simulink model "automata_learning"  (R2022a)
(part 6 of 10)

0.1781599223613739 * x2 - 0.022882848978042603) - 1.0) / (exp(0.6783225536346436 * x1 + 0.1781599223613739 * x2 - 0.022882848978042603) + 1.0) + 0.600735068321228 * (exp(0.485967755317688 * x2 - 1.1853820085525513 * x1 + 0.018565522506833076) - 1.0) / (exp(0.485967755317688 * x2 - 1.1853820085525513 * x1 + 0.018565522506833076) + 1.0) + 0.07953598350286484 * (exp(1.4361170530319214 * x1 - 0.5143741369247437 * x2 + 0.003782355459406972) - 1.0) / (exp(1.4361170530319214 * x1 - 0.5143741369247437 * x2 + 0.003782355459406972) + 1.0) - 0.3439609110355377 * (exp(1.0996636152267456 * x1 - 0.4135805368423462 * x2 + 0.20608894526958466) - 1.0) / (exp(1.0996636152267456 * x1 - 0.4135805368423462 * x2 + 0.20608894526958466) + 1.0) - 0.26753464341163635 * (exp(1.101186752319336 * x1 + 0.23448167741298676 * x2 - 0.7151159048080444) - 1.0) / (exp(1.101186752319336 * x1 + 0.23448167741298676 * x2 - 0.7151159048080444) + 1.0) - 0.33746933937072754 * (exp(0.2064213752746582 * x1 + 0.17808765172958374 * x2 - 0.17820464074611664) - 1.0) / (exp(0.2064213752746582 * x1 + 0.17808765172958374 * x2 - 0.17820464074611664) + 1.0) + 0.7188074588775635 * (exp(0.8331294059753418 * x1 + 0.364244282245636 * x2 - 0.19144871830940247) - 1.0) / (exp(0.8331294059753418 * x1 + 0.364244282245636 * x2 - 0.19144871830940247) + 1.0) + 0.48850470781326294 * (exp(0.4359053075313568 * x1 + 0.912689745426178 * x2 + 0.2776009142398834) - 1.0) / (exp(0.4359053075313568 * x1 + 0.912689745426178 * x2 + 0.2776009142398834) + 1.0) - 0.3132037818431854 * (exp(0.4313433766365051 * x1 + 0.24489279091358185 * x2 - 0.033217817544937134) - 1.0) / (exp(0.4313433766365051 * x1 + 0.24489279091358185 * x2 - 0.033217817544937134) + 1.0) + 0.5981374979019165 * (exp(0.3509118854999542 * x1 - 0.9669473171234131 * x2 + 0.38815683126449585) - 1.0) / (exp(0.3509118854999542 * x1 - 0.9669473171234131 * x2 + 0.38815683126449585) + 1.0) + 0.47281572222709656 * (exp(0.8456477522850037 * x1 - 0.048582736402750015 * x2 + 0.05466446280479431) - 1.0) / (exp(0.8456477522850037 * x1 - 0.048582736402750015 * x2 + 0.05466446280479431) + 1.0) - 0.7066691517829895 * (exp(0.37150701880455017 * x1 - 0.23563559353351593 * x2 + 0.41328972578048706) - 1.0) / (exp(0.37150701880455017 * x1 - 0.23563559353351593 * x2 + 0.41328972578048706) + 1.0) - 0.5022667050361633 * (exp(1.5675164461135864 * x1 + 0.05015593022108078 * x2 + 0.23397907614707947) - 1.0) / (exp(1.5675164461135864 * x1 + 0.05015593022108078 * x2 + 0.23397907614707947) + 1.0) + 0.6585901379585266 * (exp(0.66331547498703 * x1 + 0.4469437301158905 * x2 + 0.06243124231696129) - 1.0) / (exp(0.66331547498703 * x1 + 0.4469437301158905 * x2 + 0.06243124231696129) + 1.0) + 0.12011811137199402) + 1.0) - 0.2208395153284073 * (exp(0.36608901619911194 * (exp(0.8134481906890869 * x1 + 0.9884344339370728 * x2 - 0.4219200313091278) - 1.0) / (exp(0.8134481906890869 * x1 + 0.9884344339370728 * x2 - 0.4219200313091278) + 1.0) - 0.7763866186141968 * (exp(0.4392474293708801 * x1 - 0.48300591111183167 * x2 + 0.1989256739616394) - 1.0) / (exp(0.4392474293708801 * x1 - 0.48300591111183167 * x2 + 0.1989256739616394) + 1.0) + 0.3814668357372284 * (exp(0.047009728848934174 * x2 - 1.010794997215271 * x1 + 0.010623830370604992) - 1.0) / (exp(0.047009728848934174 * x2 - 1.010794997215271 * x1 + 0.010623830370604992) + 1.0) + 0.550957977771759 * (exp(0.8894705772399902 * x1 - 1.0577815771102905 * x2 + 0.6941524744033813) - 1.0) / (exp(0.8894705772399902 * x1 - 1.0577815771102905 * x2 + 0.6941524744033813) + 1.0) - 0.42258381843566895 * (exp(0.8751505613327026 * x1 + 0.041782353073358536 * x2 + 0.14423272013664246) - 1.0) / (exp(0.8751505613327026 * x1 + 0.041782353073358536 * x2 + 0.14423272013664246) + 1.0) - 0.33416351675987244 * (exp(0.1809358298778534 * x2 - 1.0878992080688477 * x1 + 0.21376754343509674) - 1.0) / (exp(0.1809358298778534 * x2 - 1.0878992080688477 * x1 + 0.21376754343509674) + 1.0) - 0.5293717384338379 * (exp(0.6783225536346436 * x1 + 0.1781599223613739 * x2 - 0.022882848978042603) - 1.0) / (exp(0.6783225536346436 * x1 + 0.1781599223613739 * x2 - 0.022882848978042603) + 1.0) + 0.16978411376476288 * (exp(0.485967755317688 * x2 - 1.1853820085525513 * x1 + 0.018565522506833076) - 1.0) / (exp(0.485967755317688 * x2 - 1.1853820085525513 * x1 + 0.018565522506833076) + 1.0) - 0.07960239797830582 * (exp(1.4361170530319214 * x1 - 0.5143741369247437 * x2 + 0.003782355459406972) - 1.0) / (exp(1.4361170530319214 * x1 - 0.5143741369247437 * x2 + 0.003782355459406972) + 1.0) + 0.3012309670448303 * (exp(1.0996636152267456 * x1 - 0.4135805368423462 * x2 + 0.20608894526958466) - 1.0) / (exp(1.0996636152267456 * x1 - 0.4135805368423462 * x2 + 0.20608894526958466) + 1.0) + 0.001827016705647111 * (exp(1.101186752319336 * x1 + 0.23448167741298676 * x2 - 0.7151159048080444) - 1.0) / (exp(1.101186752319336 * x1 + 0.23448167741298676 * x2 - 0.7151159048080444) + 1.0) + 0.6800966262817383 * (exp(0.2064213752746582 * x1 + 0.17808765172958374 * x2 - 0.17820464074611664) - 1.0) / (exp(0.2064213752746582 * x1 + 0.17808765172958374 * x2 - 0.17820464074611664) + 1.0) + 0.3445820212364197 * (exp(0.8331294059753418 * x1 + 0.364244282245636 * x2 - 0.19144871830940247) - 1.0) / (exp(0.8331294059753418 * x1 + 0.364244282245636 * x2 - 0.19144871830940247) + 1.0) + 0.33697742223739624 * (exp(0.4359053075313568 * x1 + 0.912689745426178 * x2 + 0.2776009142398834) - 1.0) / (exp(0.4359053075313568 * x1 + 0.912689745426178 * x2 + 0.2776009142398834) + 1.0) + 0.6987252831459045 * (exp(0.4313433766365051 * x1 + 0.24489279091358185 * x2 - 0.033217817544937134) - 1.0) / (exp(0.4313433766365051 * x1 + 0.24489279091358185 * x2 - 0.033217817544937134) + 1.0) - 0.700903058052063 * (exp(0.3509118854999542 * x1 - 0.9669473171234131 * x2 + 0.38815683126449585) - 1.0) / (exp(0.3509118854999542 * x1 - 0.9669473171234131 * x2 + 0.38815683126449585) + 1.0) - 0.48154786229133606 * (exp(0.8456477522850037 * x1 - 0.048582736402750015 * x2 + 0.05466446280479431) - 1.0) / (exp(0.8456477522850037 * x1 - 0.048582736402750015 * x2 + 0.05466446280479431) + 1.0) - 0.6501414775848389 * (exp(0.37150701880455017 * x1 - 0.23563559353351593 * x2 + 0.41328972578048706) - 1.0) / (exp(0.37150701880455017 * x1 - 0.23563559353351593 * x2 + 0.41328972578048706) + 1.0) - 0.5015138387680054 * (exp(1.5675164461135864 * x1 + 0.05015593022108078 * x2 + 0.23397907614707947) - 1.0) / (exp(1.5675164461135864 * x1 + 0.05015593022108078 * x2 + 0.23397907614707947) + 1.0) - 0.13284653425216675 * (exp(0.66331547498703 * x1 + 0.4469437301158905 * x2 + 0.06243124231696129) - 1.0) / (exp(0.66331547498703 * x1 + 0.4469437301158905 * x2 + 0.06243124231696129) + 1.0) + 0.036147914826869965) - 1.0) / (exp(0.36608901619911194 * (exp(0.8134481906890869 * x1 + 0.9884344339370728 * x2 - 0.4219200313091278) - 1.0) / (exp(0.8134481906890869 * x1 + 0.9884344339370728 * x2 - 0.4219200313091278) + 1.0) - 0.7763866186141968 * (exp(0.4392474293708801 * x1 - 0.48300591111183167 * x2 + 0.1989256739616394) - 1.0) / (exp(0.4392474293708801 * x1 - 0.48300591111183167 * x2 + 0.1989256739616394) + 1.0) + 0.3814668357372284 * (exp(0.047009728848934174 * x2 - 1.010794997215271 * x1 + 0.010623830370604992) - 1.0) / (exp(0.047009728848934174 * x2 - 1.010794997215271 * x1 + 0.010623830370604992) + 1.0) + 0.550957977771759 * (exp(0.8894705772399902 * x1 - 1.0577815771102905 * x2 + 0.6941524744033813) - 1.0) / (exp(0.8894705772399902 * x1 - 1.0577815771102905 * x2 + 0.6941524744033813) + 1.0) - 0.42258381843566895 * (exp(0.8751505613327026 * x1 + 0.041782353073358536 * x2 + 0.14423272013664246) - 1.0) / (exp(0.8751505613327026 * x1 + 0.041782353073358536 * x2 + 0.14423272013664246) + 1.0) - 0.33416351675987244 * (exp(0.1809358298778534 * x2 - 1.0878992080688477 * x1 + 0.21376754343509674) - 1.0) / (exp(0.1809358298778534 * x2 - 1.0878992080688477 * x1 + 0.21376754343509674) + 1.0) - 0.5293717384338379 * (exp(0.6783225536346436 * x1 + 0.1781599223613739 * x2 - 0.022882848978042603) - 1.0) / (exp(0.6783225536346436 * x1 + 0.1781599223613739 * x2 - 0.022882848978042603) + 1.0) + 0.16978411376476288 * (exp(0.485967755317688 * x2 - 1.1853820085525513 * x1 + 0.018565522506833076) - 1.0) / (exp(0.485967755317688 * x2 - 1.1853820085525513 * x1 + 0.018565522506833076) + 1.0) - 0.07960239797830582 * (exp(1.4361170530319214 * x1 - 0.5143741369247437 * x2 + 0.003782355459406972) - 1.0) / (exp(1.4361170530319214 * x1 - 0.5143741369247437 * x2 + 0.003782355459406972) + 1.0) + 0.3012309670448303 * (exp(1.0996636152267456 * x1 - 0.4135805368423462 * x2 + 0.20608894526958466) - 1.0) / (exp(1.0996636152267456 * x1 - 0.4135805368423462 * x2 + 0.20608894526958466) + 1.0) + 0.001827016705647111 * (exp(1.101186752319336 * x1 + 0.23448167741298676 * x2 - 0.7151159048080444) - 1.0) / (exp(1.101186752319336 * x1 + 0.23448167741298676 * x2 - 0.7151159048080444) + 1.0) + 0.6800966262817383 * (exp(0.2064213752746582 * x1 + 0.17808765172958374 * x2 - 0.17820464074611664) - 1.0) / (exp(0.2064213752746582 * x1 + 0.17808765172958374 * x2 - 0.17820464074611664) + 1.0) + 0.3445820212364197 * (exp(0.8331294059753418 * x1 + 0.364244282245636 * x2 - 0.19144871830940247) - 1.0) / (exp(0.8331294059753418 * x1 + 0.364244282245636 * x2 - 0.19144871830940247) + 1.0) + 0.33697742223739624 * (exp(0.4359053075313568 * x1 + 0.912689745426178 * x2 + 0.2776009142398834) - 1.0) / (exp(0.4359053075313568 * x1 + 0.912689745426178 * x2 + 0.2776009142398834) + 1.0) + 0.6987252831459045 * (exp(0.4313433766365051 * x1 + 0.24489279091358185 * x2 - 0.033217817544937134) - 1.0) / (exp(0.4313433766365051 * x1 + 0.24489279091358185 * x2 - 0.033217817544937134) + 1.0) - 0.700903058052063 * (exp(0.3509118854999542 * x1 - 0.9669473171234131 * x2 + 0.38815683126449585) - 1.0) / (exp(0.3509118854999542 * x1 - 0.9669473171234131 * x2 + 0.38815683126449585) + 1.0) - 0.48154786229133606 * (exp(0.8456477522850037 * x1 - 0.048582736402750015 * x2 + 0.05466446280479431) - 1.0) / (exp(0.8456477522850037 * x1 - 0.048582736402750015 * x2 + 0.05466446280479431) + 1.0) - 0.6501414775848389 * (exp(0.37150701880455017 * x1 - 0.23563559353351593 * x2 + 0.41328972578048706) - 1.0) / (exp(0.37150701880455017 * x1 - 0.23563559353351593 * x2 + 0.41328972578048706) + 1.0) - 0.5015138387680054 * (exp(1.5675164461135864 * x1 + 0.05015593022108078 * x2 + 0.23397907614707947) - 1.0) / (exp(1.5675164461135864 * x1 + 0.05015593022108078 * x2 + 0.23397907614707947) + 1.0) - 0.13284653425216675 * (exp(0.66331547498703 * x1 + 0.4469437301158905 * x2 + 0.06243124231696129) - 1.0) / (exp(0.66331547498703 * x1 + 0.4469437301158905 * x2 + 0.06243124231696129) + 1.0) + 0.036147914826869965) + 1.0) + 0.5369366407394409 * (exp(0.41898313164711 * (exp(0.4392474293708801 * x1 - 0.48300591111183167 * x2 + 0.1989256739616394) - 1.0) / (exp(0.4392474293708801 * x1 - 0.48300591111183167 * x2 + 0.1989256739616394) + 1.0) + 0.5099337100982666 * (exp(0.8134481906890869 * x1 + 0.9884344339370728 * x2 - 0.4219200313091278) - 1.0) / (exp(0.8134481906890869 * x1 + 0.9884344339370728 * x2 - 0.4219200313091278) + 1.0) - 0.1566210687160492 * (exp(0.047009728848934174 * x2 - 1.010794997215271 * x1 + 0.010623830370604992) - 1.0) / (exp(0.047009728848934174 * x2 - 1.010794997215271 * x1 + 0.010623830370604992) + 1.0) + 0.6093736886978149 * (exp(0.8894705772399902 * x1 - 1.0577815771102905 * x2 + 0.6941524744033813) - 1.0) / (exp(0.8894705772399902 * x1 - 1.0577815771102905 * x2 + 0.6941524744033813) + 1.0) - 0.6370351910591125 * (exp(0.8751505613327026 * x1 + 0.041782353073358536 * x2 + 0.14423272013664246) - 1.0) / (exp(0.8751505613327026 * x1 + 0.041782353073358536 * x2 + 0.14423272013664246) + 1.0) + 0.0998457819223404 * (exp(0.1809358298778534 * x2 - 1.0878992080688477 * x1 + 0.21376754343509674) - 1.0) / (exp(0.1809358298778534 * x2 - 1.0878992080688477 * x1 + 0.21376754343509674) + 1.0) + 0.7771844863891602 * (exp(0.6783225536346436 * x1 + 0.1781599223613739 * x2 - 0.022882848978042603) - 1.0) / (exp(0.6783225536346436 * x1 + 0.1781599223613739 * x2 - 0.022882848978042603) + 1.0) + 0.7646798491477966 * (exp(0.485967755317688 * x2 - 1.1853820085525513 * x1 + 0.018565522506833076) - 1.0) / (exp(0.485967755317688 * x2 - 1.1853820085525513 * x1 + 0.018565522506833076) + 1.0) - 0.14706474542617798 * (exp(1.4361170530319214 * x1 - 0.5143741369247437 * x2 + 0.003782355459406972) - 1.0) / (exp(1.4361170530319214 * x1 - 0.5143741369247437 * x2 + 0.003782355459406972) + 1.0) + 0.44270166754722595 * (exp(1.0996636152267456 * x1 - 0.4135805368423462 * x2 + 0.20608894526958466) - 1.0) / (exp(1.0996636152267456 * x1 - 0.4135805368423462 * x2 + 0.20608894526958466) + 1.0) + 0.05599430948495865 * (exp(1.101186752319336 * x1 + 0.23448167741298676 * x2 - 0.7151159048080444) - 1.0) / (exp(1.101186752319336 * x1 + 0.23448167741298676 * x2 - 0.7151159048080444) + 1.0) - 0.4630465507507324 * (exp(0.2064213752746582 * x1 + 0.17808765172958374 * x2 - 0.17820464074611664) - 1.0) / (exp(0.2064213752746582 * x1 + 0.17808765172958374 * x2 - 0.17820464074611664) + 1.0) + 0.8380157351493835 * (exp(0.8331294059753418 * x1 + 0.364244282245636 * x2 - 0.19144871830940247) - 1.0) / (exp(0.8331294059753418 * x1 + 0.364244282245636 * x2 - 0.19144871830940247) + 1.0) + 0.12685304880142212 * (exp(0.4359053075313568 * x1 + 0.912689745426178 * x2 + 0.2776009142398834) - 1.0) / (exp(0.4359053075313568 * x1 + 0.912689745426178 * x2 + 0.2776009142398834) + 1.0) - 0.704443097114563 * (exp(0.4313433766365051 * x1 + 0.24489279091358185 * x2 - 0.033217817544937134) - 1.0) / (exp(0.4313433766365051 * x1 + 0.24489279091358185 * x2 - 0.033217817544937134) + 1.0) + 0.23543411493301392 * (exp(0.3509118854999542 * x1 - 0.9669473171234131 * x2 + 0.38815683126449585) - 1.0) / (exp(0.3509118854999542 * x1 - 0.9669473171234131 * x2 + 0.38815683126449585) + 1.0) - 0.16425514221191406 * (exp(0.8456477522850037 * x1 - 0.048582736402750015 * x2 + 0.05466446280479431) - 1.0) / (exp(0.8456477522850037 * x1 - 0.048582736402750015 * x2 + 0.05466446280479431) + 1.0) + 0.33761852979660034 * (exp(0.37150701880455017 * x1 - 0.23563559353351593 * x2 + 0.41328972578048706) - 1.0) / (exp(0.37150701880455017 * x1 - 0.23563559353351593 * x2 + 0.41328972578048706) + 1.0) - 0.23770417273044586 * (exp(1.5675164461135864 * x1 + 0.05015593022108078 * x2 + 0.23397907614707947) - 1.0) / (exp(1.5675164461135864 * x1 + 0.05015593022108078 * x2 + 0.23397907614707947) + 1.0) + 0.6810302138328552 * (exp(0.66331547498703 * x1 + 0.4469437301158905 * x2 + 0.06243124231696129) - 1.0) / (exp(0.66331547498703 * x1 + 0.4469437301158905 * x2 + 0.06243124231696129) + 1.0) + 0.16052111983299255) - 1.0) / (exp(0.41898313164711 * (exp(0.4392474293708801 * x1 - 0.48300591111183167 * x2 + 0.1989256739616394) - 1.0) / (exp(0.4392474293708801 * x1 - 0.48300591111183167 * x2 + 0.1989256739616394) + 1.0) + 0.5099337100982666 * (exp(0.8134481906890869 * x1 + 0.9884344339370728 * x2 - 0.4219200313091278) - 1.0) / (exp(0.8134481906890869 * x1 + 0.9884344339370728 * x2 - 0.4219200313091278) + 1.0) - 0.1566210687160492 * (exp(0.047009728848934174 * x2 - 1.010794997215271 * x1 + 0.010623830370604992) - 1.0) / (exp(0.047009728848934174 * x2 - 1.010794997215271 * x1 + 0.010623830370604992) + 1.0) + 0.6093736886978149 * (exp(0.8894705772399902 * x1 - 1.0577815771102905 * x2 + 0.6941524744033813) - 1.0) / (exp(0.8894705772399902 * x1 - 1.0577815771102905 * x2 + 0.6941524744033813) + 1.0) - 0.6370351910591125 * (exp(0.8751505613327026 * x1 + 0.041782353073358536 * x2 + 0.14423272013664246) - 1.0) / (exp(0.8751505613327026 * x1 + 0.041782353073358536 * x2 + 0.14423272013664246) + 1.0) + 0.0998457819223404 * (exp(0.1809358298778534 * x2 - 1.0878992080688477 * x1 + 0.21376754343509674) - 1.0) / (exp(0.1809358298778534 * x2 - 1.0878992080688477 * x1 + 0.21376754343509674) + 1.0) + 0.7771844863891602 * (exp(0.6783225536346436 * x1 + 0.1781599223613739 * x2 - 0.022882848978042603) - 1.0) / (exp(0.6783225536346436 * x1 + 0.1781599223613739 * x2 - 0.022882848978042603) + 1.0) + 0.7646798491477966 * (exp(0.485967755317688 * x2 - 1.1853820085525513 * x1 + 0.018565522506833076) - 1.0) / (exp(0.485967755317688 * x2 - 1.1853820085525513 * x1 + 0.018565522506833076) + 1.0) - 0.14706474542617798 * (exp(1.4361170530319214 * x1 - 0.5143741369247437 * x2 + 0.003782355459406972) - 1.0) / (exp(1.4361170530319214 * x1 - 0.5143741369247437 * x2 + 0.003782355459406972) + 1.0) + 0.44270166754722595 * (exp(1.0996636152267456 * x1 - 0.4135805368423462 * x2 + 0.20608894526958466) - 1.0) / (exp(1.0996636152267456 * x1 - 0.4135805368423462 * x2 + 0.20608894526958466) + 1.0) + 0.05599430948495865 * (exp(1.101186752319336 * x1 + 0.23448167741298676 * x2 - 0.7151159048080444) - 1.0) / (exp(1.101186752319336 * x1 + 0.23448167741298676 * x2 - 0.7151159048080444) + 1.0) - 0.4630465507507324 * (exp(0.2064213752746582 * x1 + 0.17808765172958374 * x2 - 0.17820464074611664) - 1.0) / (exp(0.2064213752746582 * x1 + 0.17808765172958374 * x2 - 0.17820464074611664) + 1.0) + 0.8380157351493835 * (exp(0.8331294059753418 * x1 + 0.364244282245636 * x2 - 0.19144871830940247) - 1.0) / (exp(0.8331294059753418 * x1 + 0.364244282245636 * x2 - 0.19144871830940247) + 1.0) + 0.12685304880142212 * (exp(0.4359053075313568 * x1 + 0.912689745426178 * x2 + 0.2776009142398834) - 1.0) / (exp(0.4359053075313568 * x1 + 0.912689745426178 * x2 + 0.2776009142398834) + 1.0) - 0.704443097114563 * (exp(0.4313433766365051 * x1 + 0.24489279091358185 * x2 - 0.033217817544937134) - 1.0) / (exp(0.4313433766365051 * x1 + 0.24489279091358185 * x2 - 0.033217817544937134) + 1.0) + 0.23543411493301392 * (exp(0.3509118854999542 * x1 - 0.9669473171234131 * x2 + 0.38815683126449585) - 1.0) / (exp(0.3509118854999542 * x1 - 0.9669473171234131 * x2 + 0.38815683126449585) + 1.0) - 0.16425514221191406 * (exp(0.8456477522850037 * x1 - 0.048582736402750015 * x2 + 0.05466446280479431) - 1.0) / (exp(0.8456477522850037 * x1 - 0.048582736402750015 * x2 + 0.05466446280479431) + 1.0) + 0.33761852979660034 * (exp(0.37150701880455017 * x1 - 0.23563559353351593 * x2 + 0.41328972578048706) - 1.0) / (exp(0.37150701880455017 * x1 - 0.23563559353351593 * x2 + 0.41328972578048706) + 1.0) - 0.23770417273044586 * (exp(1.5675164461135864 * x1 + 0.05015593022108078 * x2 + 0.23397907614707947) - 1.0) / (exp(1.5675164461135864 * x1 + 0.05015593022108078 * x2 + 0.23397907614707947) + 1.0) + 0.6810302138328552 * (exp(0.66331547498703 * x1 + 0.4469437301158905 * x2 + 0.06243124231696129) - 1.0) / (exp(0.66331547498703 * x1 + 0.4469437301158905 * x2 + 0.06243124231696129) + 1.0) + 0.16052111983299255) + 1.0) + 0.13662315905094147;
    x1_out=x1;
    x2_out=x2;
    automata_learning_location =1;
  state loc2
    du:
